simulink subsystem "SignalSwitch"  (R2020b)
settings: Solver=VariableStepAuto  StartTime=0.0  StopTime=10.0  RelTol=1e-3
libraries: simulink x2
settings Model: Creator=PaulWintz  LastModifiedBy=PaulWintz

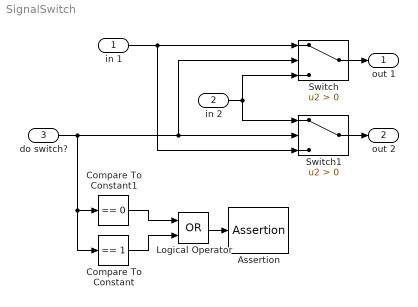
== system SignalSwitch ==
  in 1 : Inport
  in 2 : Inport  Port=2
  do switch? : Inport  Port=3
  Assertion : Assertion
  Compare To Constant : simulink/Logic and Bit Operations/Compare To Constant  relop===  const=1  OutDataTypeStr=boolean
  Compare To Constant1 : simulink/Logic and Bit Operations/Compare To Constant  relop===  const=0  OutDataTypeStr=boolean
  Logical Operator : Logic  Operator=OR  AllPortsSameDT=off  OutDataTypeStr=boolean
  Switch : Switch  Criteria=u2 > Threshold
  Switch1 : Switch  Criteria=u2 > Threshold
  out 1 : Outport
  out 2 : Outport  Port=2
  wires:
  Switch/1 -> out 1/1
  in 1/1 -> Switch1/3, Switch/1
  in 2/1 -> Switch1/1, Switch/3
  Switch1/1 -> out 2/1
  do switch?/1 -> Compare To Constant1/1, Compare To Constant/1, Switch1/2, Switch/2
  Logical Operator/1 -> Assertion/1
  Compare To Constant/1 -> Logical Operator/2
  Compare To Constant1/1 -> Logical Operator/1
